simulink model "ex1_s"  (R2021b)
settings: Solver=VariableStepAuto  StartTime=0.0  StopTime=10.0  RelTol=1e-3
undefined symbols (not defined in the file or in its folder): A, B, C

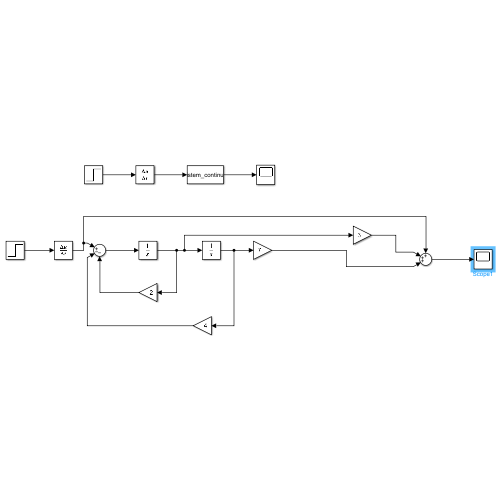
[thumbnail: Simulink's stored preview of the top-level diagram]
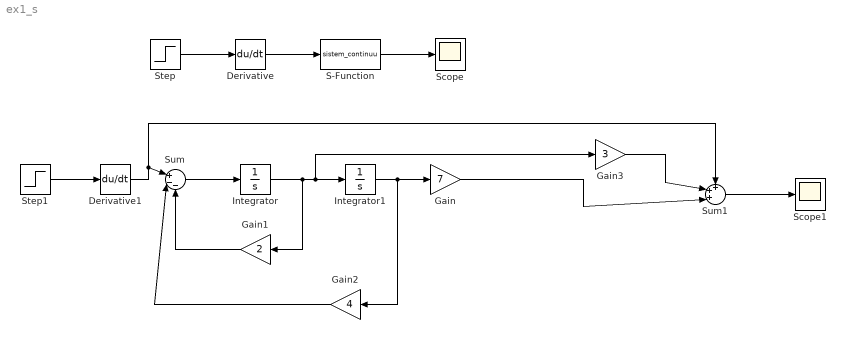
== system ex1_s ==
  Derivative : Derivative
  Derivative1 : Derivative
  Gain : Gain  Gain=7
  Gain1 : Gain  Gain=2
  Gain2 : Gain  Gain=4
  Gain3 : Gain  Gain=3
  Integrator : Integrator
  Integrator1 : Integrator
  S-Function : S-Function  FunctionName=sistem_continuu  Parameters=A,B,C  SFunctionDeploymentMode=off  EnableBusSupport=off
  Scope : Scope
  Scope1 : Scope
  Step : Step  SampleTime=0
  Step1 : Step  SampleTime=0
  Sum : Sum  Inputs=|+--
  Sum1 : Sum  Inputs=+++|
  wires:
  Step/1 -> Derivative/1
  Derivative/1 -> S-Function/1
  S-Function/1 -> Scope/1
  Gain2/1 -> Sum/2
  Step1/1 -> Derivative1/1
  Derivative1/1 -> Sum1/1, Sum/1
  Sum/1 -> Integrator/1
  Sum1/1 -> Scope1/1
  Integrator/1 -> Gain1/1, Gain3/1, Integrator1/1
  Gain1/1 -> Sum/3
  Integrator1/1 -> Gain2/1, Gain/1
  Gain/1 -> Sum1/3
  Gain3/1 -> Sum1/2
